simulink model "EPSmotor"  (R2019b)
settings: Solver=VariableStepAuto  StartTime=0.0  StopTime=10.0  RelTol=1e-3
undefined symbols (not defined in the file or in its folder): Moment_limit, Steering_Angle, Vehicle_Speed
libraries: powerlib x7, simulink x1, eePwmGenerator x1
settings Model: Creator=DUY  LastModifiedBy=DUY

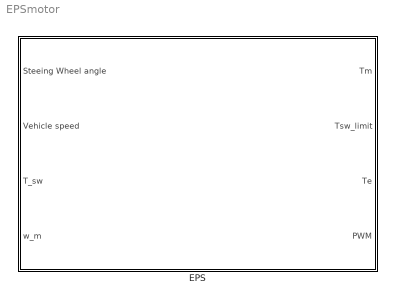
== system EPSmotor ==
  EPS : Subsystem

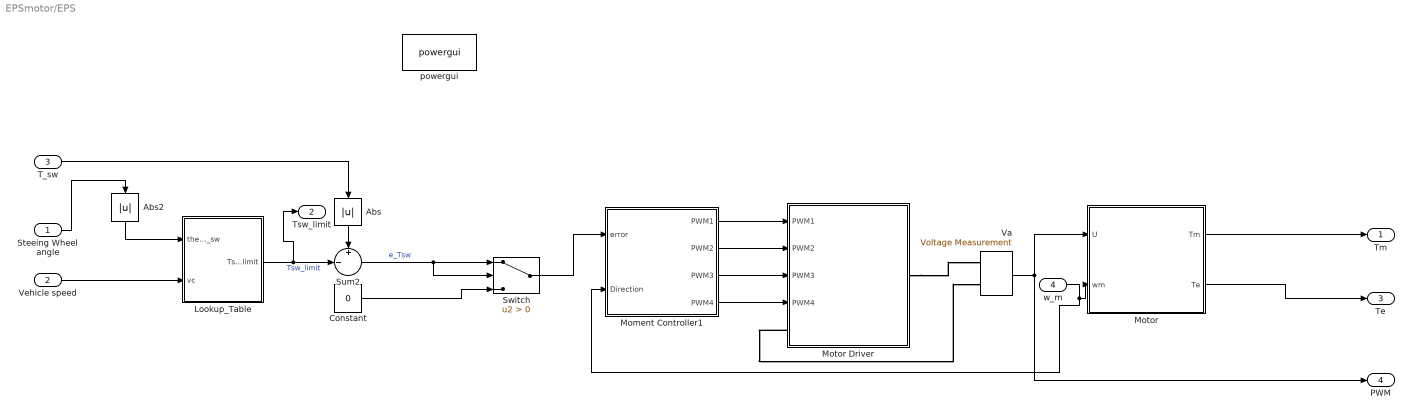
== system EPSmotor/EPS ==
  Steeing Wheel angle : Inport
  Vehicle speed : Inport  Port=2
  T_sw : Inport  Port=3
  w_m : Inport  Port=4
  Abs : Abs
  Abs2 : Abs
  Constant : Constant  Value=0
  Lookup_Table : Subsystem
  Moment Controller1 : Subsystem
  "Motor " : Subsystem  mask{Km=0.456, Kb=0.3533, B=0.071, J=0.00218907, L=0.002, R=0.6}
      mask prompts: Km "Torque constant"; Kb "Back emf constant"; B "Viscous friction"; J "Inertia"; L "Inductance"; R "Resistance"
      mask Display: image('motor.png');
  Motor Driver : Subsystem
      mask Display: image('bridge.png');
  Sum2 : Sum  Inputs=+|-||
  Switch : Switch  Criteria=u2 > Threshold
  Va : powerlib/Measurements/Voltage Measurement  Tag=PoWeRsYsTeMmEaSuReMeNt  PhasorSimulation=off  OutputType=Magnitude  PSBequivalent=0
  powergui : powerlib/powergui  Priority=1  SimulationMode=Discrete  SampleTime=0.0001  frequency=60  Iterations=50  frequencyindice=0  Pbase=100e6  ErrMax=1e-4  UnitsV=kV  UnitsW=MW  buscounter=0  FunctionMessages=off  echomessages=off  EnableUseOfTLC=off  CurrentSourceSwitches=off  DisableSnubberDevices=off  DisableRonSwitches=off  DisableVfSwitches=off  DisplayEquations=off  AutomaticDiscreteSolvers=off  SolverType=Tustin/Backward Euler (TBE)  Interpol=off  ExternalGateDelay=off  methode=off  Ts=100  x0status=blocks  SPID=on  SwTol=0  HookPort=off  NonlinearTolerance=1e-4  nMaxIteration=100  ContinueOnMaxIteration=off  RestoreLinks=warning  ResistiveCurrentMeasurement=off  Frange=[0:2:500]  Ylog=off  Xlog=on  ShowGrid=off  save=off  variable=ZData  structure=0  ZoomFFT=off  StartTime=0.0  cycles=1  DisplayStyle=1  fundamental=60  FreqAxis=off  MaxFrequency=1000  frequencyindicesteady=1  RmsSteady=1  display=off
      settings: SourceProductName=Simscape Electrical
  Tm : Outport  VectorParamsAs1DForOutWhenUnconnected=off
  Tsw_limit : Outport  Port=2  VectorParamsAs1DForOutWhenUnconnected=off
  Te : Outport  Port=3  VectorParamsAs1DForOutWhenUnconnected=off
  PWM : Outport  Port=4  VectorParamsAs1DForOutWhenUnconnected=off
  wires:
  Abs2/1 -> Lookup_Table/1(theta_sw)
  Moment Controller1/1(PWM1) -> Motor Driver/1(PWM1)
  Moment Controller1/4(PWM4) -> Motor Driver/4(PWM4)
  Switch/1 -> Moment Controller1/1(error)
  T_sw/1 -> Abs/1
  Moment Controller1/2(PWM2) -> Motor Driver/2(PWM2)
  Steeing Wheel angle/1 -> Abs2/1
  Moment Controller1/3(PWM3) -> Motor Driver/3(PWM3)
  w_m/1 -> "Motor "/2(wm), Moment Controller1/2(Direction)
  Va/1 -> "Motor "/1(U), PWM/1
  Sum2/1 -> Switch/2, Switch/1  "e_Tsw"
  Constant/1 -> Switch/3
  Abs/1 -> Sum2/1
  "Motor "/2(Te) -> Te/1
  "Motor "/1(Tm) -> Tm/1
  Vehicle speed/1 -> Lookup_Table/2(vc)
  Lookup_Table/1(Tsw_limit) -> Sum2/2, Tsw_limit/1  "Tsw_limit"
  connections:
  Motor Driver/LConn1 -- Va/LConn2
  Motor Driver/RConn1 -- Va/LConn1

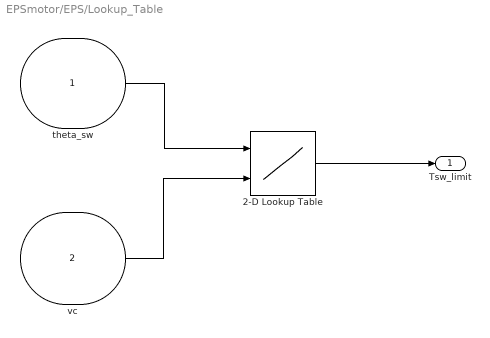
== system EPSmotor/EPS/Lookup_Table ==
  theta_sw : Inport
      mask Display: image('1.png');
  vc : Inport  Port=2
      mask Display: image('speed.png');
  2-D Lookup Table : Lookup_n-D  BreakpointsForDimension1=Steering_Angle  BreakpointsForDimension2=Vehicle_Speed  Table=Moment_limit  InternalRulePriority=Speed  RndMeth=Simplest  InputSameDT=on
  Tsw_limit : Outport  VectorParamsAs1DForOutWhenUnconnected=off
  wires:
  theta_sw/1 -> 2-D Lookup Table/1
  vc/1 -> 2-D Lookup Table/2
  2-D Lookup Table/1 -> Tsw_limit/1

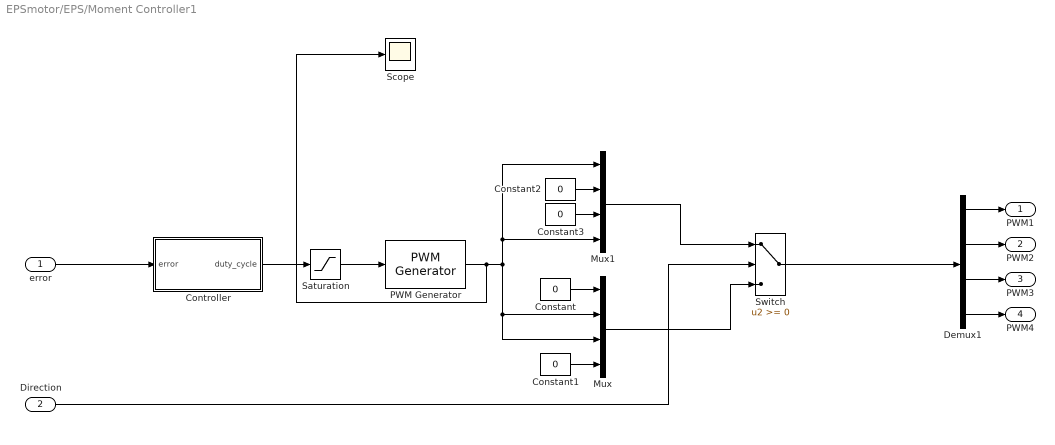
== system EPSmotor/EPS/Moment Controller1 ==
  error : Inport
  Direction : Inport  Port=2
  Constant{,1..3} (4 alike) : Constant  Value=0
  Controller : Subsystem
  Demux1 : Demux
  Mux : Mux
  Mux1 : Mux
  PWM Generator : eePwmGenerator/PWM Generator  CarrCount=Up  Tper=0.0001  Ts=0.00001
      settings: SourceProductName=Simscape Electrical
  Saturation : Saturate  UpperLimit=1  LowerLimit=0
  Scope : Scope
  Switch : Switch
  PWM1 : Outport  VectorParamsAs1DForOutWhenUnconnected=off
  PWM2 : Outport  Port=2  VectorParamsAs1DForOutWhenUnconnected=off
  PWM3 : Outport  Port=3  VectorParamsAs1DForOutWhenUnconnected=off
  PWM4 : Outport  Port=4  VectorParamsAs1DForOutWhenUnconnected=off
  wires:
  Demux1/1 -> PWM1/1
  Demux1/4 -> PWM4/1
  Demux1/3 -> PWM3/1
  Demux1/2 -> PWM2/1
  Mux1/1 -> Switch/1
  Mux/1 -> Switch/3
  Switch/1 -> Demux1/1
  Constant2/1 -> Mux1/2
  Constant3/1 -> Mux1/3
  Constant/1 -> Mux/1
  Constant1/1 -> Mux/4
  Controller/1(duty_cycle) -> Saturation/1
  PWM Generator/1 -> Scope/1, Mux/2, Mux/3, Mux1/1, Mux1/4
  Saturation/1 -> PWM Generator/1
  Direction/1 -> Switch/2
  error/1 -> Controller/1(error)

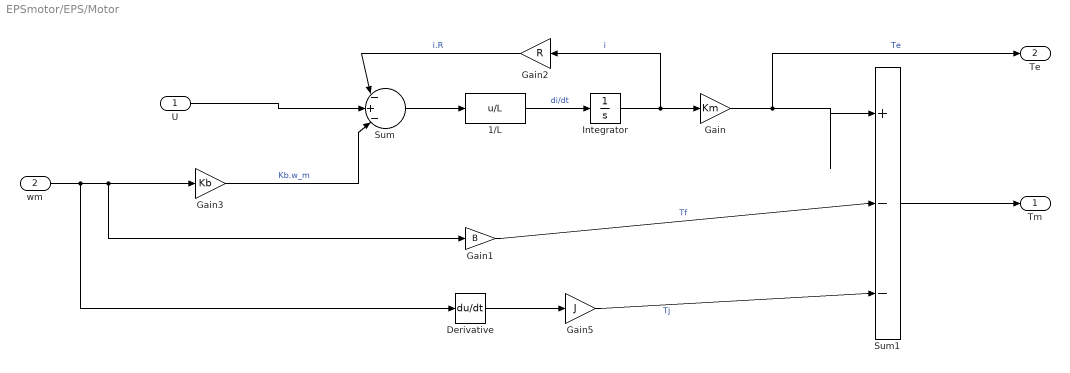
== system EPSmotor/EPS/Motor  ==
  U : Inport
  wm : Inport  Port=2
  1/L : Fcn  Expr=u/L
  Derivative : Derivative
  Gain : Gain  Gain=Km
  Gain1 : Gain  Gain=B
  Gain2 : Gain  Gain=R
  Gain3 : Gain  Gain=Kb
  Gain5 : Gain  Gain=J
  Integrator : Integrator
  Sum : Sum  Inputs=|-+-|
  Sum1 : Sum  Inputs=|+--
  Tm : Outport  VectorParamsAs1DForOutWhenUnconnected=off
  Te : Outport  Port=2  VectorParamsAs1DForOutWhenUnconnected=off
  wires:
  Sum/1 -> 1/L/1
  1/L/1 -> Integrator/1  "di/dt"
  Integrator/1 -> Gain2/1, Gain/1  "i"
  Gain/1 -> Te/1, Sum1/1  "Te"
  Gain2/1 -> Sum/1  "i.R"
  Gain1/1 -> Sum1/2  "Tf"
  Sum1/1 -> Tm/1
  Derivative/1 -> Gain5/1
  Gain5/1 -> Sum1/3  "Tj"
  wm/1 -> Derivative/1, Gain1/1, Gain3/1
  U/1 -> Sum/2
  Gain3/1 -> Sum/3  "Kb.w_m"

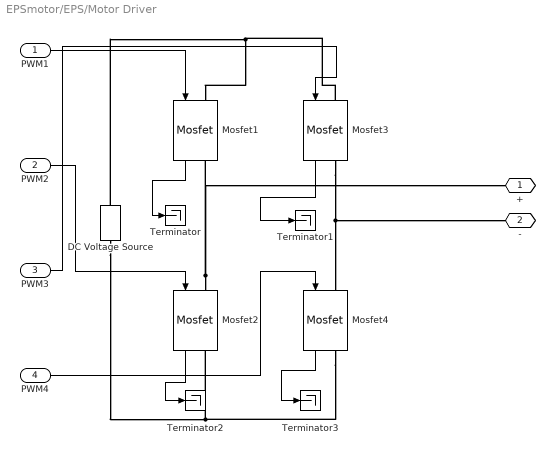
== system EPSmotor/EPS/Motor Driver ==
  PWM1 : Inport
  PWM2 : Inport  Port=2
  PWM3 : Inport  Port=3
  PWM4 : Inport  Port=4
  DC Voltage Source : powerlib/Electrical Sources/DC Voltage Source  Amplitude=36  Measurements=Voltage
  Mosfet{1..4} (4 alike) : powerlib/Power Electronics/Mosfet  Ron=0.1  Lon=0  Rd=0.01  Vfd=0  IC=0  Rs=1e5  Cs=inf  Measurements=on
  Terminator{,1..3} (4 alike) : Terminator
  + : PMIOPort  Side=Right
  - : PMIOPort  Port=2  Side=Left
  wires:
  PWM3/1 -> Mosfet3/1
  PWM1/1 -> Mosfet1/1
  PWM2/1 -> Mosfet2/1
  PWM4/1 -> Mosfet4/1
  Mosfet1/1 -> Terminator/1
  Mosfet3/1 -> Terminator1/1
  Mosfet2/1 -> Terminator2/1
  Mosfet4/1 -> Terminator3/1
  connections:
  Mosfet4/RConn1 -- DC Voltage Source/LConn1 -- Mosfet2/RConn1
  Mosfet2/LConn1 -- Mosfet1/RConn1 -- +/RConn1
  Mosfet3/LConn1 -- DC Voltage Source/RConn1 -- Mosfet1/LConn1
  Mosfet3/RConn1 -- -/RConn1 -- Mosfet4/LConn1

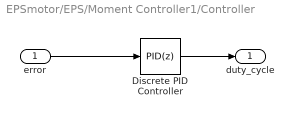
== system EPSmotor/EPS/Moment Controller1/Controller ==
  error : Inport
  Discrete PID Controller : simulink/Continuous/PID Controller  Controller=PID  Form=Parallel  TimeDomain=Discrete-time  SampleTime=-1  IntegratorMethod=Forward Euler  FilterMethod=Forward Euler  ControllerParametersSource=internal  P=5  I=0.2  D=0  UseFilter=on  N=100  TunerSelectOption=Frequency Response Based  InitialConditionSource=internal  InitialConditionForIntegrator=0  InitialConditionForFilter=0  DifferentiatorICPrevScaledInput=0  ExternalReset=none  TrackingMode=off  Kt=1  LimitOutput=on  UpperSaturationLimit=1  LowerSaturationLimit=0  LinearizeAsGain=off  AntiWindupMode=back-calculation  Kb=1  POutMin=[]  POutMax=[]  IOutMin=[]  IOutMax=[]  DOutMin=[]  DOutMax=[]  NOutMin=[]  NOutMax=[]  SumOutMin=[]  SumOutMax=[]  SaturationOutMin=[]  SaturationOutMax=[]  PParamMin=[]  PParamMax=[]  IParamMin=[]  IParamMax=[]  DParamMin=[]  DParamMax=[]  NParamMin=[]  NParamMax=[]  KbParamMin=[]  KbParamMax=[]  KtParamMin=[]  KtParamMax=[]  KbOutMin=[]  KbOutMax=[]  KtOutMin=[]  KtOutMax=[]  IntegratorOutMin=[]  IntegratorOutMax=[]  FilterOutMin=[]  FilterOutMax=[]  SumI1OutMin=[]  SumI1OutMax=[]  SumI2OutMin=[]  SumI2OutMax=[]  SumI3OutMin=[]  SumI3OutMax=[]  SumI4OutMin=[]  SumI4OutMax=[]  SumDOutMin=[]  SumDOutMax=[]  DifferentiatorOutMin=[]  DifferentiatorOutMax=[]  FilterDiffOutCoefMin=[]  FilterDiffOutCoefMax=[]  ReciprocalOutMin=[]  ReciprocalOutMax=[]  SumDenOutMin=[]  SumDenOutMax=[]  SumNumOutMin=[]  SumNumOutMax=[]  DivideOutMin=[]  DivideOutMax=[]  IntegratorContinuousStateAttributes=''  IntegratorStateMustResolveToSignalObject=off  IntegratorRTWStateStorageClass=Auto  FilterContinuousStateAttributes=''  FilterStateMustResolveToSignalObject=off  FilterRTWStateStorageClass=Auto  ParallelPVariant=InternalParameters  IdealPVariant=Disabled  IVariant=InternalParameters  DVariant=InternalParameters  IntegratorVariant=Discrete  SatVariant=Enabled  AWVariant=BackCalculation  PCopyVariant=Disabled  TRVariant=Disabled  FdbkBlocksVariant=Forward  IdealPFdbkVariant=Disabled  SatFdbkVariant=Disabled  DerivativeFilterVariant=ForwardEulerFilter  NVariant=InternalParameters  NCopyVariant=Disabled  FilterICVariant=InternalICsFilter  IntegratorICVariant=InternalICs  ExternalResetVariant=Disabled  TRSumVariant=Passthrough  SumFdbkVariant=Disabled  SumVariant=Sum_PID
  duty_cycle : Outport
  wires:
  Discrete PID Controller/1 -> duty_cycle/1
  error/1 -> Discrete PID Controller/1
